simulink model "Swingup_mpc"  (R2021b)
settings: Solver=ode1  StartTime=0.0  StopTime=120  RelTol=1e-3  EnableMultiTasking=on
values from neighbouring files (symbols this model uses):
  A_aug = [str_discr_sys.A,str_discr_sys.B ... (first row only)    [Controller_Dashboard.m]    (also in MPC_controller.m; MPC_controller_testing.m; max_structure_MPC_controller_testing.m)
  B_aug = [str_discr_sys.B;0]    [Controller_Dashboard.m]    (also in MPC_controller.m; MPC_controller_testing.m; max_structure_MPC_controller_testing.m)
  C_aug = [str_discr_sys.C, zeros(2,1)]    [Controller_Dashboard.m]    (also in MPC_controller.m; MPC_controller_testing.m; max_structure_MPC_controller_testing.m)
  D_aug = str_discr_sys.D    [Controller_Dashboard.m]    (also in MPC_controller.m; MPC_controller_testing.m; max_structure_MPC_controller_testing.m)
  epsilon = 0.00242    [Controller_Dashboard.m]    (also in MPC_controller.m; MPC_controller_testing.m; max_structure_MPC_controller_testing.m)
  Extr_states = [eye(4),zeros(4,1)]    [Controller_Dashboard.m]    (also in MPC_controller.m; MPC_controller_testing.m; max_structure_MPC_controller_testing.m)
  g = 9.81    [Controller_Dashboard.m]
  h = 0.01    [Controller_Dashboard.m]    (also in Design_of_nonlinear_controller.m = g4*D*alpha - g3*D*theta; MPC_controller.m; MPC_controller_testing.m; max_structure_MPC_controller_testing.m)
  Jp = mp*Lp^2/3    (= 0.000133128)    [Controller_Dashboard.m]
  ke = 0.15    [Controller_Dashboard.m]
  kt = 0.042    [Controller_Dashboard.m]
  Kw = [0,0,0,0,1]    [Controller_Dashboard.m]    (also in MPC_controller.m; MPC_controller_testing.m; max_structure_MPC_controller_testing.m)
  l = Lp/2    (= 0.0645)    [Controller_Dashboard.m]
  mp = 0.024    [Controller_Dashboard.m]
  mr = 0.095    [Controller_Dashboard.m]
  r = 0.085    [Controller_Dashboard.m]
  Rk = 1e-9    (= 1e-09)    [Controller_Dashboard.m]    (also in MPC_controller.m; MPC_controller_testing.m = 1e-12; max_structure_MPC_controller_testing.m = 1e-12)
  Rm = 8.4    [Controller_Dashboard.m]
  u_max = 10    [Controller_Dashboard.m]
undefined symbols (not defined in the file or in its folder): Discrete, Humusoft, MF634, Time
libraries: simulink x3, sldrtlib x2, ctrlSharedLib x1, simulink_extras x1
settings Model: Creator=rbabuska  LastModifiedBy=wpanijhuis
settings SolverCC: AlgebraicLoopSolver=TrustRegion
settings DataIOCC: LimitDataPoints=on  SaveFormat=Array  SignalLoggingSaveFormat=ModelDataLogs  ReturnWorkspaceOutputs=off
settings OptimizationCC: ExpressionDepthLimit=2147483647  LifeSpan=inf
settings DebuggingCC: UnderspecifiedInitializationDetection=Classic  MergeDetectMultiDrivingBlocksExec=none  FcnCallInpInsideContextMsg=warning  StateNameClashWarn=warning  SFUnexpectedBacktrackingDiag=warning  SFNoUnconditionalDefaultTransitionDiag=warning  SFExecutionAtInitializationDiag=none  SFMachineParentedDataDiag=warning  ArithmeticOperatorsInVariantConditions=warning
settings HardwareCC: ProdBitPerPointer=32  ProdBitPerSizeT=32  ProdBitPerPtrDiffT=32  ProdLargestAtomicFloat=None  ProdIntDivRoundTo=Undefined  ProdEndianess=Unspecified  ProdWordSize=32  ProdHWDeviceType=32-bit Generic
settings ModelReferenceCC: PropagateSignalLabelsOutOfModel=off
settings SFSimCC: SimUseLocalCustomCode=off  CustomCodeUndefinedFunction=UseInterfaceOnly
settings RTWCC: RTWUseLocalCustomCode=off
settings CodeAppCC: StateflowObjectComments=on
settings GRTTargetCC: TargetLangStandard=C89/C90 (ANSI)  CombineOutputUpdateFcns=off  GRTInterface=on
settings ConfigComp: CovMetricSettings=dw  CovSaveCumulativeToWorkspaceVar=on  CovSaveSingleToWorkspaceVar=on  CovExternalEMLEnable=off  CovSFcnEnable=off

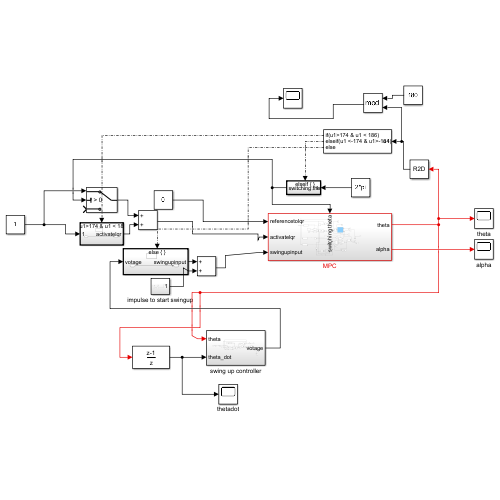
[thumbnail: Simulink's stored preview of the top-level diagram]
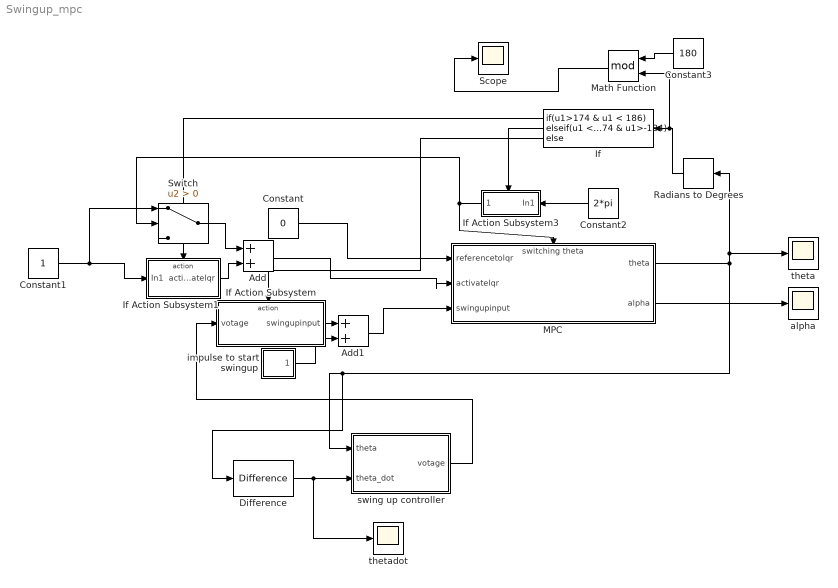
== system Swingup_mpc ==
  Add : Sum
  Add1 : Sum
  Constant : Constant  Value=0
  Constant1 : Constant
  Constant2 : Constant  Value=2*pi
  Constant3 : Constant  Value=180
  Difference : simulink/Discrete/Difference  ICPrevInput=0.0  OutMin=[]  OutMax=[]  OutDataType=fixdt(1, 16)  OutScaling=2^-10  DoSatur=off
  If : If  IfExpression=u1>174 & u1 < 186  ElseIfExpressions=u1 <-174 & u1>-184
  If Action Subsystem : Subsystem  TreatAsAtomicUnit=on
  If Action Subsystem1 : Subsystem  TreatAsAtomicUnit=on
  If Action Subsystem3 : Subsystem  TreatAsAtomicUnit=on
  MPC : Subsystem
      settings: PortSchema="{\"entries\":[{\"content\":{\"sides\":[{\"content\":{\"connectorIds\":[\"In1\",\"In2\",\"In3\"]},\"type\":\"ConnectorPlacement.EquallySpacedRectSide\",\"uuid\":\"9db084a4-f3e8-4cdd-afd7-80f171250afb\"},{\"content\":{\"connectorIds\":[\"Out1\",\"Out2\"],\"side\":\"RIGHT\"},\"type\":\"ConnectorPlacement.EquallySpacedRectSide\",\"uuid\":\"2cad91b5-cf79-4872-a768-f1b673626e3c\"},{\"content\":{\"connectorIds\":[\"In4\"],\"side\":\"TOP\"},\"type\":\"ConnectorPlacement.EquallySpacedRectSide\",\"uuid\":\"043f2d69-1466-4c8d-8cce-e26869681d3b\"}]},\"type\":\"ConnectorPlacement.EquallySpacedConnector\",\"uuid\":\"e19d8d99-f04f-4830-94fe-43bf442ec7a8\"}],\"packageUris\":[\"http://schema.mathworks.com/mf0/Connector/R2020b\"],\"version\":\"1.0\"}"
  Math Function : Math  Operator=mod  SaturateOnIntegerOverflow=on
  Radians to Degrees : simulink_extras/Transformations/Radians to Degrees
  Scope : Scope
  Switch : Switch  Criteria=u2 > Threshold
  alpha : Scope
  impulse to start swingup : Subsystem
  swing up controller : Subsystem
  theta : Scope
  thetadot : Scope
  wires:
  Constant/1 -> MPC/1(referencetolqr)
  MPC/1(theta) -> Difference/1, swing up controller/1(theta), Radians to Degrees/1, theta/1
  Difference/1 -> thetadot/1, swing up controller/2(theta_dot)
  Radians to Degrees/1 -> Math Function/2, If/1
  If/3 -> If Action Subsystem/Action
  Constant1/1 -> If Action Subsystem1/1(In1), Switch/1
  Add/1 -> MPC/2(activatelqr)
  Add1/1 -> MPC/3(swingupinput)
  swing up controller/1(votage) -> If Action Subsystem/1(votage)
  If Action Subsystem/1(swingupinput) -> Add1/1
  impulse to start swingup/1(Out1) -> Add1/2
  If/2 -> If Action Subsystem3/Action
  If/1 -> If Action Subsystem1/Action
  Switch/1 -> Add/1
  If Action Subsystem1/1(activatelqr) -> Add/2
  Constant2/1 -> If Action Subsystem3/1(In1)
  If Action Subsystem3/1(switching theta) -> Switch/2, MPC/4(switching theta)
  MPC/2(alpha) -> alpha/1
  Constant3/1 -> Math Function/1
  Math Function/1 -> Scope/1

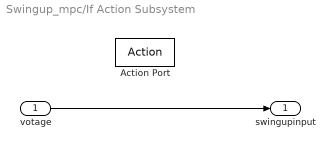
== system Swingup_mpc/If Action Subsystem ==
  votage : Inport
  Action Port : ActionPort  ActionPortLabel=else
  swingupinput : Outport
  wires:
  votage/1 -> swingupinput/1

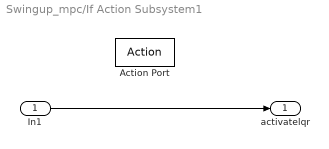
== system Swingup_mpc/If Action Subsystem1 ==
  In1 : Inport
  Action Port : ActionPort  ActionPortLabel=if(u1>174 & u1 < 186)
  activatelqr : Outport
  wires:
  In1/1 -> activatelqr/1

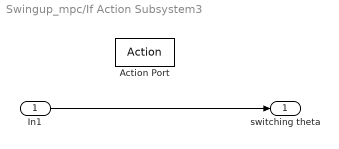
== system Swingup_mpc/If Action Subsystem3 ==
  In1 : Inport
  Action Port : ActionPort  ActionPortLabel=elseif(u1 <-174 & u1>-184)
  switching theta : Outport
  wires:
  In1/1 -> switching theta/1

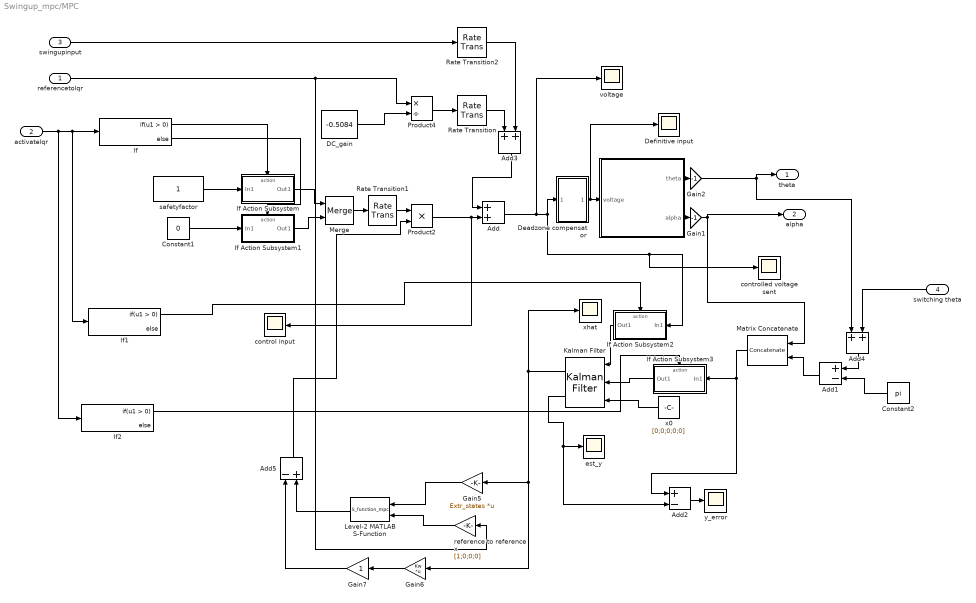
== system Swingup_mpc/MPC ==
  referencetolqr : Inport
  activatelqr : Inport  Port=2
  swingupinput : Inport  Port=3
  switching theta : Inport  Port=4
  " " : Subsystem  LoadFcn=hwinit  InitFcn=hwinit  mask{h=h}
      mask prompts: h "Sampling period [s]"
      mask Display:
      | disp('Qube-Servo')
      | port_label('output',1,'theta')
      | port_label('output',2,'alpha')
      | port_label('input',1,'V')
  Add : Sum  RndMeth=Nearest
  Add1 : Sum  Inputs=+-
  Add2 : Sum  Inputs=+-
  Add3 : Sum
  Add4 : Sum
  Add5 : Sum  Inputs=-+
  Constant1 : Constant  Value=0
  Constant2 : Constant  Value=pi
  DC_gain : Constant  Value=-0.5084  SampleTime=h
  Deadzone compensator : Subsystem
  Definitive input : Scope
  Gain1 : Gain  Gain=-1
  Gain2 : Gain  Gain=-1
  Gain5 : Gain  Gain=Extr_states  Multiplication=Matrix(K*u)
  Gain6 : Gain  Gain=Kw  Multiplication=Matrix(K*u)
  Gain7 : Gain
  If : If
  If Action Subsystem : Subsystem  TreatAsAtomicUnit=on
  If Action Subsystem1 : Subsystem  TreatAsAtomicUnit=on
  If Action Subsystem2 : Subsystem  TreatAsAtomicUnit=on
  If Action Subsystem3 : Subsystem  TreatAsAtomicUnit=on
  If1 : If
  If2 : If
  Kalman Filter : ctrlSharedLib/Kalman Filter  TimeDomain=Discrete-Time  UseCurrentEstimator=on  ModelSource=Individual A, B, C, D matrices  ModelSourceVariable=ss(0.95,1,1,0,1)  A=A_aug  B=B_aug  C=C_aug  D=D_aug  NumberOfStates=1  NumberOfInputs=1  NumberOfOutputs=1  InitialEstimateSource=Input port  X0=0  P0=10  UseK=off  UseGH=off  NumberOfProcessNoiseInputs=1  G=1  TimeInvariantG=on  H=0  TimeInvariantH=on  Q=Qk  TimeInvariantQ=on  R=Rk  TimeInvariantR=on  N=0  TimeInvariantN=on  AddInputPort=on  AddEnablePort=off  OutputEstimatedY=on  OutputP=off  Ts=h
  Level-2 MATLAB S-Function : M-S-Function  FunctionName=S_function_mpc  Parameters=fast_opt
  Matrix Concatenate : Concatenate  ConcatenateDimension=2
  Merge : Merge
  Product2 : Product
  Product4 : Product  Inputs=*/
  Rate Transition : RateTransition  OutPortSampleTime=h
  Rate Transition1 : RateTransition  OutPortSampleTime=h
  Rate Transition2 : RateTransition  OutPortSampleTime=h
  control input : Scope
  controlled voltage sent : Scope
  est_y : Scope
  reference to reference x : Gain  Gain=[1;0;0;0]
  safetyfactor : Constant  SampleTime=h
  voltage : Scope
  x0 : Constant  Value=[0;0;0;0;0]
  xhat : Scope
  y_error : Scope
  theta : Outport
  alpha : Outport  Port=2
  wires:
  Matrix Concatenate/1 -> If Action Subsystem3/1(In1), Add2/1
  Add/1 -> voltage/1, Deadzone compensator/1(In1), If Action Subsystem2/1(In1), controlled voltage sent/1
  x0/1 -> Kalman Filter/3
  If/1 -> If Action Subsystem/Action
  Product4/1 -> Rate Transition/1
  If Action Subsystem/1(Out1) -> Merge/1
  Add3/1 -> Add/1
  " "/1(theta) -> Gain2/1
  Kalman Filter/2 -> Add2/2, est_y/1
  Constant2/1 -> Add1/2
  DC_gain/1 -> Product4/2
  " "/2(alpha) -> Gain1/1
  activatelqr/1 -> If2/1, If1/1, If/1
  Add2/1 -> y_error/1
  If/2 -> If Action Subsystem1/Action
  Product2/1 -> control input/1, Add/2
  Constant1/1 -> If Action Subsystem1/1(In1)
  Add5/1 -> Product2/2
  Merge/1 -> Rate Transition1/1
  Gain2/1 -> Add4/1, theta/1
  Rate Transition1/1 -> Product2/1
  safetyfactor/1 -> If Action Subsystem/1(In1)
  Deadzone compensator/1(Out1) -> Definitive input/1, " "/1(voltage)
  If Action Subsystem1/1(Out1) -> Merge/2
  Add1/1 -> Matrix Concatenate/2
  Gain1/1 -> Matrix Concatenate/1, alpha/1
  Rate Transition/1 -> Add3/1
  swingupinput/1 -> Rate Transition2/1
  Rate Transition2/1 -> Add3/2
  If Action Subsystem2/1(Out1) -> Kalman Filter/1
  If Action Subsystem3/1(Out1) -> Kalman Filter/2
  If1/1 -> If Action Subsystem2/Action
  If2/1 -> If Action Subsystem3/Action
  Add4/1 -> Add1/1
  switching theta/1 -> Add4/2
  Level-2 MATLAB S-Function/1 -> Add5/2
  Gain7/1 -> Add5/1
  reference to reference x/1 -> Level-2 MATLAB S-Function/2
  Kalman Filter/1 -> xhat/1, Gain6/1, Gain5/1
  Gain5/1 -> Level-2 MATLAB S-Function/1
  referencetolqr/1 -> Product4/1, reference to reference x/1
  Gain6/1 -> Gain7/1

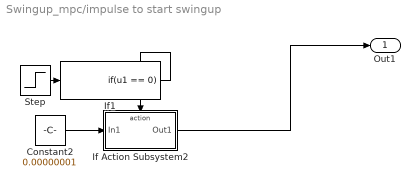
== system Swingup_mpc/impulse to start swingup ==
  Constant2 : Constant  Value=0.00000001
  If Action Subsystem2 : Subsystem  TreatAsAtomicUnit=on
  If1 : If  IfExpression=u1 == 0  ShowElse=off
  Step : Step  Time=h  SampleTime=h
  Out1 : Outport
  wires:
  Step/1 -> If1/1
  Constant2/1 -> If Action Subsystem2/1(In1)
  If1/1 -> If Action Subsystem2/Action
  If Action Subsystem2/1(Out1) -> Out1/1

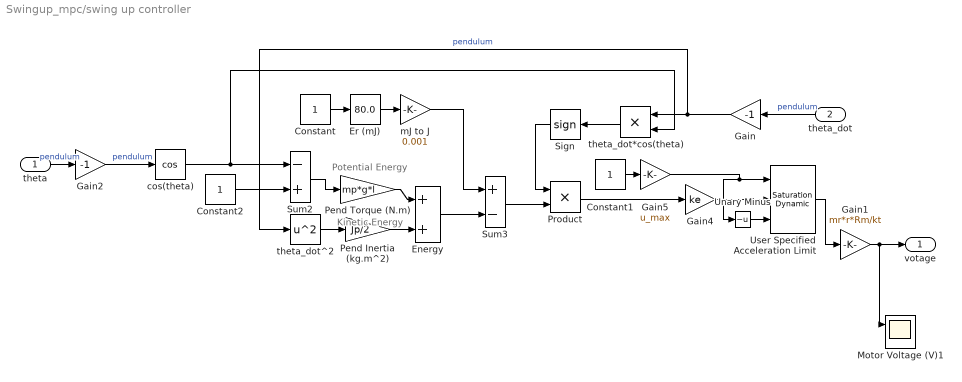
== system Swingup_mpc/swing up controller ==
  note: Kinetic Energy
  note: Potential Energy
  theta : Inport
  theta_dot : Inport  Port=2
  Constant : Constant
  Constant1 : Constant
  Constant2 : Constant
  Energy : Sum  SaturateOnIntegerOverflow=on
  Er (mJ) : simulink/Math Operations/Slider Gain  gain=80.0  low=0  high=1000
  Gain : Gain  Gain=-1
  Gain1 : Gain  Gain=mr*r*Rm/kt
  Gain2 : Gain  Gain=-1
  Gain4 : Gain  Gain=ke
  Gain5 : Gain  Gain=u_max
  Motor Voltage (V)1 : Scope  NumInputPorts=2
  Pend Inertia (kg.m^2) : Gain  Gain=Jp/2
  Pend Torque (N.m) : Gain  Gain=mp*g*l
  Product : Product  RndMeth=Zero
  Sign : Signum
  Sum2 : Sum  Inputs=-+  SaturateOnIntegerOverflow=on
  Sum3 : Sum  Inputs=+-  SaturateOnIntegerOverflow=on
  Unary Minus : UnaryMinus
  User Specified Acceleration Limit : simulink/Discontinuities/Saturation Dynamic  OutMin=-u_max  OutMax=u_max  OutDataTypeStr=Inherit: Same as second input  OutDataType=fixdt(1, 16)  OutScaling=2^-10  DoSatur=off
  cos(theta) : Trigonometry  Operator=cos
  mJ to J : Gain  Gain=0.001
  theta_dot*cos(theta) : Product  RndMeth=Zero
  theta_dot^2 : Math  Operator=square  SignedPower=on  SaturateOnIntegerOverflow=on
  votage : Outport  VectorParamsAs1DForOutWhenUnconnected=off
  wires:
  Gain5/1 -> Unary Minus/1, User Specified Acceleration Limit/1
  Constant1/1 -> Gain5/1
  Er (mJ)/1 -> mJ to J/1
  User Specified Acceleration Limit/1 -> Gain1/1
  Energy/1 -> Sum3/2
  theta_dot*cos(theta)/1 -> Sign/1
  Constant2/1 -> Sum2/2
  Sum2/1 -> Pend Torque (N.m)/1
  Pend Torque (N.m)/1 -> Energy/1
  theta_dot^2/1 -> Pend Inertia (kg.m^2)/1
  Sum3/1 -> Product/2
  Product/1 -> Gain4/1
  Gain1/1 -> Motor Voltage (V)1/1, votage/1
  Sign/1 -> Product/1
  Constant/1 -> Er (mJ)/1
  Unary Minus/1 -> User Specified Acceleration Limit/3
  Gain4/1 -> User Specified Acceleration Limit/2
  Pend Inertia (kg.m^2)/1 -> Energy/2
  mJ to J/1 -> Sum3/1
  Gain2/1 -> cos(theta)/1  "pendulum"
  cos(theta)/1 -> theta_dot*cos(theta)/2, Sum2/1
  Gain/1 -> theta_dot^2/1, theta_dot*cos(theta)/1  "pendulum"
  theta_dot/1 -> Gain/1  "pendulum"
  theta/1 -> Gain2/1  "pendulum"

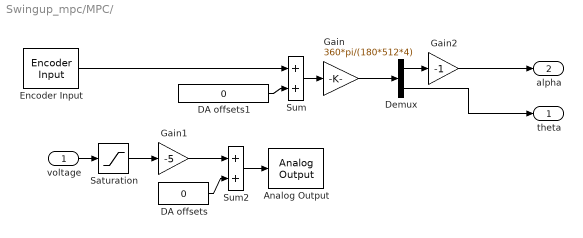
== system Swingup_mpc/MPC/  ==
  voltage : Inport
  Analog Output : sldrtlib/Analog Output  SampleTime=h  MaxMissedTicks=100  ShowMissedTicks=off  YieldWhenWaiting=off  DrvName=Humusoft/MF634  DrvAddress=4294967295  DrvOptions=0  Channels=[1]  RangeMode=2  VoltRange=1  InitialValue=0  FinalValue=0
      settings: AttributesFormatString=Humusoft\nMF634 [auto]
  DA offsets : Constant  Value=0
  DA offsets1 : Constant  Value=0  SampleTime=h
  Demux : Demux  Outputs=2
  Encoder Input : sldrtlib/Encoder Input  SampleTime=h  MaxMissedTicks=100  ShowMissedTicks=off  YieldWhenWaiting=off  DrvName=Humusoft/MF634  DrvAddress=4294967295  DrvOptions=0  Channels=[1,2]  QuadMode=3  IndexPulse=1  InputFilter=Inf  DataType=1
      settings: AttributesFormatString=Humusoft\nMF634 [auto]
  Gain : Gain  Gain=360*pi/(180*512*4)  SaturateOnIntegerOverflow=on  OutDataTypeStr=Inherit: Same as input  ParamDataTypeStr=Inherit: Same as input
  Gain1 : Gain  Gain=-5  SaturateOnIntegerOverflow=on  OutDataTypeStr=Inherit: Same as input  ParamDataTypeStr=Inherit: Same as input
  Gain2 : Gain  Gain=-1  SaturateOnIntegerOverflow=on  OutDataTypeStr=Inherit: Same as input  ParamDataTypeStr=Inherit: Same as input
  Saturation : Saturate  UpperLimit=1  LowerLimit=-1
  Sum : Sum  InputSameDT=on  SaturateOnIntegerOverflow=on  OutDataTypeStr=Inherit: Same as first input
  Sum2 : Sum  InputSameDT=on  SaturateOnIntegerOverflow=on  OutDataTypeStr=Inherit: Same as first input
  theta : Outport  Tag=Cable length
  alpha : Outport  Tag=Cable length  Port=2
  wires:
  Sum/1 -> Gain/1
  DA offsets1/1 -> Sum/2
  Gain1/1 -> Sum2/1
  Sum2/1 -> Analog Output/1
  DA offsets/1 -> Sum2/2
  voltage/1 -> Saturation/1
  Encoder Input/1 -> Sum/1
  Saturation/1 -> Gain1/1
  Demux/1 -> Gain2/1
  Gain/1 -> Demux/1
  Gain2/1 -> alpha/1
  Demux/2 -> theta/1

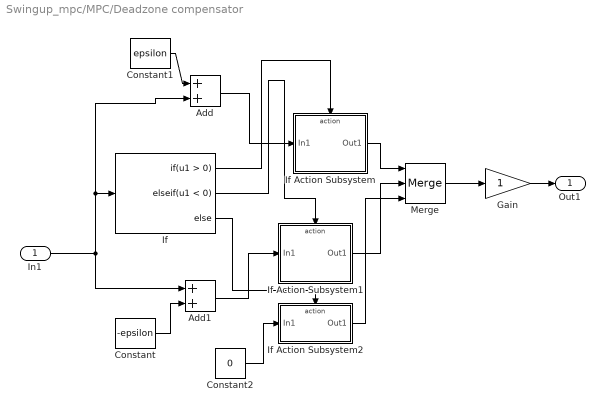
== system Swingup_mpc/MPC/Deadzone compensator ==
  In1 : Inport
  Add : Sum
  Add1 : Sum
  Constant : Constant  Value=-epsilon
  Constant1 : Constant  Value=epsilon
  Constant2 : Constant  Value=0
  Gain : Gain
  If : If  ElseIfExpressions=u1 < 0
  If Action Subsystem : Subsystem  TreatAsAtomicUnit=on
  If Action Subsystem1 : Subsystem  TreatAsAtomicUnit=on
  If Action Subsystem2 : Subsystem  TreatAsAtomicUnit=on
  Merge : Merge  Inputs=3
  Out1 : Outport
  wires:
  If Action Subsystem/1(Out1) -> Merge/1
  Gain/1 -> Out1/1
  Merge/1 -> Gain/1
  If/2 -> If Action Subsystem1/Action
  Add/1 -> If Action Subsystem/1(In1)
  If/1 -> If Action Subsystem/Action
  If Action Subsystem1/1(Out1) -> Merge/2
  In1/1 -> Add1/1, Add/2, If/1
  Constant1/1 -> Add/1
  Constant/1 -> Add1/2
  Add1/1 -> If Action Subsystem1/1(In1)
  Constant2/1 -> If Action Subsystem2/1(In1)
  If/3 -> If Action Subsystem2/Action
  If Action Subsystem2/1(Out1) -> Merge/3

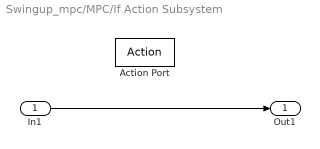
== system Swingup_mpc/MPC/If Action Subsystem ==
  In1 : Inport
  Action Port : ActionPort  ActionPortLabel=if(u1 > 0)
  Out1 : Outport
  wires:
  In1/1 -> Out1/1

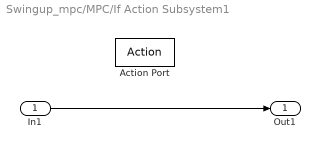
== system Swingup_mpc/MPC/If Action Subsystem1 ==
  In1 : Inport
  Action Port : ActionPort  ActionPortLabel=else
  Out1 : Outport
  wires:
  In1/1 -> Out1/1

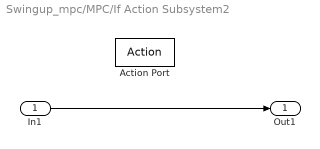
== system Swingup_mpc/MPC/If Action Subsystem2 ==
  In1 : Inport
  Action Port : ActionPort  ActionPortLabel=if(u1 > 0)
  Out1 : Outport
  wires:
  In1/1 -> Out1/1

== system Swingup_mpc/MPC/If Action Subsystem3 ==
  In1 : Inport
  Action Port : ActionPort  ActionPortLabel=if(u1 > 0)
  Out1 : Outport
  wires:
  In1/1 -> Out1/1

== system Swingup_mpc/impulse to start swingup/If Action Subsystem2 ==
  In1 : Inport
  Action Port : ActionPort  ActionPortLabel=if(u1 == 0)
  Out1 : Outport
  wires:
  In1/1 -> Out1/1

== system Swingup_mpc/MPC/Deadzone compensator/If Action Subsystem ==
  In1 : Inport
  Action Port : ActionPort  ActionPortLabel=if(u1 > 0)
  Out1 : Outport
  wires:
  In1/1 -> Out1/1

== system Swingup_mpc/MPC/Deadzone compensator/If Action Subsystem1 ==
  In1 : Inport
  Action Port : ActionPort  ActionPortLabel=elseif(u1 < 0)
  Out1 : Outport
  wires:
  In1/1 -> Out1/1

== system Swingup_mpc/MPC/Deadzone compensator/If Action Subsystem2 ==
  In1 : Inport
  Action Port : ActionPort  ActionPortLabel=else
  Out1 : Outport
  wires:
  In1/1 -> Out1/1
